simulink model "pendulum"  (Simulink 5.0)
settings: Solver=ode45  StartTime=0.00  StopTime=15  FixedStep=0.1  MaxStep=0.001  RelTol=1e-3
values from neighbouring files (symbols this model uses):
  K = [0 K]    [Pendulum_init.m]
libraries: vrlib x1
CloseFcn:
  | rtwprivate ssgencode ModelCloseRequest pendsim
settings Model: LastModifiedBy=Gato  RTWOptions="-aEnforceIntegerDowncast=1 -aExtMode=0 -aExtModeTesting=0 -aFoldNonRolledExpr=1 -aForceParamTrailComments=0 -aGenerateComments=1 -aGenerateReport=0 -aIgnoreCustomStorageClasses=1 -aIncDataTypeInIds=0 -aIncHierarchyInIds=0 -aInlineInvariantSignals=0 -aInlinedPrmAccess=\"Literals\" -aLocalBlockOutputs=1 -aLogVarNameModifier=\"rt_\" -aMaxRTWIdLen=31 -aPrefixModelToSubsysFcnNames=1 -aRTWVerbose=1 -aRollThreshold=5 -aShowEliminatedStatements=0"

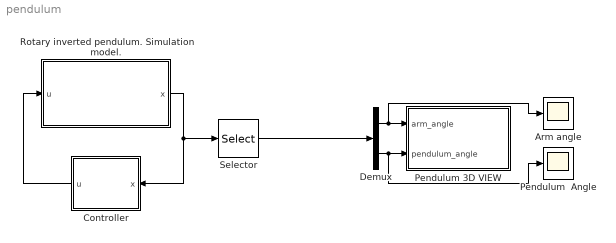
== system pendulum ==
  Arm angle : Scope
  Controller : Subsystem  Orientation=left
  Demux : Demux  Outputs=2
  Pendulum  Angle : Scope
  Pendulum 3D VIEW : Subsystem  TreatAsAtomicUnit=on
  Rotary inverted pendulum. Simulation model. : Subsystem  TreatAsAtomicUnit=on  mask{l=0.5, m1=1, b1=0.4, r=1, m2=0.5, b2=0.1, x1_0=0, x2_0=0, x3_0=0.1, x4_0=0, g=9.81}
      mask prompts: l "Arm length [m]"; m1 "Arm mass [kg]"; b1 "Arm dumping coefficient"; r "Pendulum lenght [m]"; m2 "Pendulum mass [kg]"; b2 "Pendulum dumping coefficient"; x1_0 "Arm initial angle [rad]"; x2_0 "Arm initial speed [m/s]"; x3_0 "Pendulum initial angle [rad]"; x4_0 "Pendulum initial speed [m/s]"; g "Gravity"
  Selector : Selector  Elements=[1 3]  InputPortWidth=4
  wires:
  Demux/1 -> Pendulum 3D VIEW/1(arm_angle), Arm angle/1
  Demux/2 -> Pendulum 3D VIEW/2(pendulum_angle), Pendulum  Angle/1
  Selector/1 -> Demux/1
  Rotary inverted pendulum. Simulation model./1(x) -> Selector/1, Controller/1(x)
  Controller/1(u) -> Rotary inverted pendulum. Simulation model./1(u)

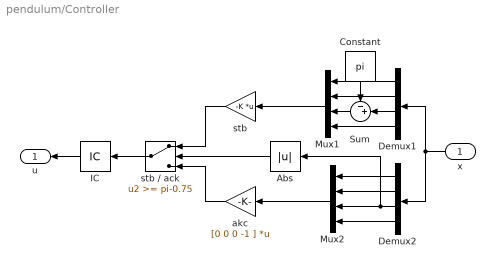
== system pendulum/Controller ==
  x : Inport  Orientation=left
  Abs : Abs  Orientation=left  SaturateOnIntegerOverflow=on
  Constant : Constant  Orientation=down  Value=pi
  Demux1 : Demux  Orientation=left
  Demux2 : Demux  Orientation=left
  IC : InitialCondition  Orientation=left  Value=0
  Mux1 : Mux  Orientation=left
  Mux2 : Mux  Orientation=left
  Sum : Sum  Orientation=left  Inputs=-+|  SaturateOnIntegerOverflow=on
  akc : Gain  Orientation=left  Gain=[0 0 0 -1 ]  Multiplication=Matrix(K*u)  SaturateOnIntegerOverflow=on
  stb : Gain  Orientation=left  Gain=-K  Multiplication=Matrix(K*u)  SaturateOnIntegerOverflow=on
  stb / ack : Switch  Orientation=left  Threshold=pi-0.75  SaturateOnIntegerOverflow=on
  u : Outport  Orientation=left
  wires:
  Demux2/2 -> Mux2/2
  Demux2/4 -> Mux2/4
  Demux2/1 -> Mux2/1
  Demux2/3 -> Mux2/3, Abs/1
  Mux2/1 -> akc/1
  IC/1 -> u/1
  Demux1/2 -> Mux1/2
  Demux1/1 -> Mux1/1
  stb/1 -> stb / ack/1
  Demux1/3 -> Sum/2
  Constant/1 -> Sum/1
  Sum/1 -> Mux1/3
  Mux1/1 -> stb/1
  Demux1/4 -> Mux1/4
  x/1 -> Demux1/1, Demux2/1
  akc/1 -> stb / ack/3
  Abs/1 -> stb / ack/2
  stb / ack/1 -> IC/1

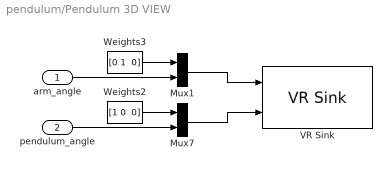
== system pendulum/Pendulum 3D VIEW ==
  arm_angle : Inport
  pendulum_angle : Inport  Port=2
  Mux1 : Mux  Inputs=2
  Mux7 : Mux  Inputs=2
  VR Sink : vrlib/VR Sink  SampleTime=0.1  ViewEnable=on  RemoteChange=off  RemoteView=off  FieldsWritten=Arm.rotation.4#Pendulum.rotation.4  WorldFileName=pendulum_vr.WRL  WorldDescription=pendulum_vr  AutoView=on  FigureProperties="{'Position', 'Name', 'Viewpoint', 'CameraBound', 'CameraDirection', 'CameraPosition', 'CameraUpVector', 'ZoomFactor', 'Antialiasing', 'Headlight', 'Lighting', 'PanelMode', 'Textures', 'Transparency', 'Wireframe', 'NavZones', 'InfoStrip', 'NavMode', 'NavSpeed', ; [9.0000000000000000e+000  2.5000000000000000e+001  6.5400000000000000e+002  9.6500000000000000e+002], 'pendulum_vr', '', 'on', [0.0000000000000000e+000  0.0000000000000000e+000 -1.0000000000000000e+000], [0.0000000000000000e+000  0.0000000000000000e+000  1.0000000000000000e+001], [0.0000000000000000e+000  1.0000000000000000e+000  0.0000000000000000e+000], [1.0000000000000000e+000], 'off', 'on', 'on', 'opaque', 'on', 'on', 'off', 'off', 'off', 'fly', 'normal', ; }"
  Weights2 : Constant  Value="[1 0  0]"
  Weights3 : Constant  Value="[0 1  0]"
  wires:
  Weights2/1 -> Mux7/1
  Mux7/1 -> VR Sink/2
  pendulum_angle/1 -> Mux7/2
  Weights3/1 -> Mux1/1
  Mux1/1 -> VR Sink/1
  arm_angle/1 -> Mux1/2

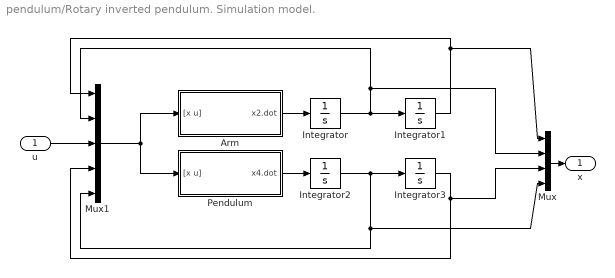
== system pendulum/Rotary inverted pendulum. Simulation model. ==
  u : Inport
  Arm : Subsystem  TreatAsAtomicUnit=on
  Integrator : Integrator  InitialCondition=x2_0
  Integrator1 : Integrator  InitialCondition=x1_0
  Integrator2 : Integrator  InitialCondition=x4_0
  Integrator3 : Integrator  InitialCondition=x3_0
  Mux : Mux
  Mux1 : Mux  Inputs=5
  Pendulum : Subsystem  TreatAsAtomicUnit=on
  x : Outport
  wires:
  Integrator3/1 -> Mux1/4, Mux/3
  Integrator2/1 -> Integrator3/1, Mux1/5, Mux/4
  Integrator/1 -> Integrator1/1, Mux1/2, Mux/2
  Pendulum/1(x4.dot) -> Integrator2/1
  Arm/1(x2.dot) -> Integrator/1
  Mux1/1 -> Pendulum/1("[x u]"), Arm/1("[x u]")
  u/1 -> Mux1/3
  Integrator1/1 -> Mux1/1, Mux/1
  Mux/1 -> x/1

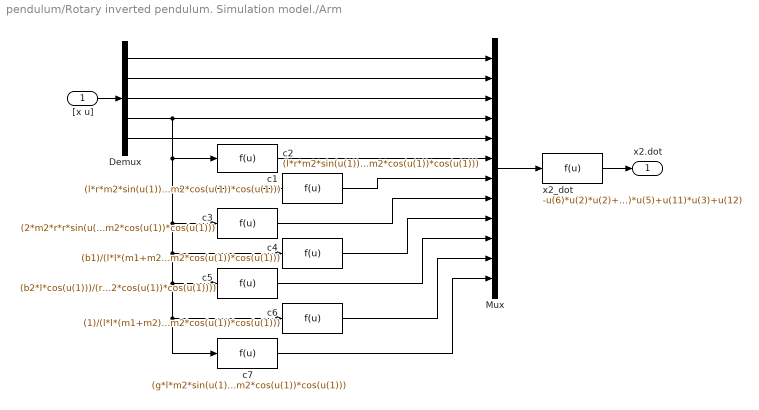
== system pendulum/Rotary inverted pendulum. Simulation model./Arm ==
  "[x u]" : Inport
  Demux : Demux  Outputs=5
  Mux : Mux  Inputs=12
  c1 : Fcn  Expr=(l*r*m2*sin(u(1))*cos(u(1))*cos(u(1)))/(l*l*(m1+m2)+r*r*m2*sin(u(1))*sin(u(1))-l*l*m2*cos(u(1))*cos(u(1)))
  c2 : Fcn  Expr=(l*r*m2*sin(u(1)))/(l*l*(m1+m2)+r*r*m2*sin(u(1))*sin(u(1))-l*l*m2*cos(u(1))*cos(u(1)))
  c3 : Fcn  Expr=(2*m2*r*r*sin(u(1))*cos(u(1)))/(l*l*(m1+m2)+r*r*m2*sin(u(1))*sin(u(1))-l*l*m2*cos(u(1))*cos(u(1)))
  c4 : Fcn  Expr=(b1)/(l*l*(m1+m2)+r*r*m2*sin(u(1))*sin(u(1))-l*l*m2*cos(u(1))*cos(u(1)))
  c5 : Fcn  Expr=(b2*l*cos(u(1)))/(r*(l*l*(m1+m2)+r*r*m2*sin(u(1))*sin(u(1))-l*l*m2*cos(u(1))*cos(u(1))))
  c6 : Fcn  Expr=(1)/(l*l*(m1+m2)+r*r*m2*sin(u(1))*sin(u(1))-l*l*m2*cos(u(1))*cos(u(1)))
  c7 : Fcn  Expr=(g*l*m2*sin(u(1))*cos(u(1)))/(l*l*(m1+m2)+r*r*m2*sin(u(1))*sin(u(1))-l*l*m2*cos(u(1))*cos(u(1)))
  x2_dot : Fcn  Expr=-u(6)*u(2)*u(2)+u(7)*u(5)*u(5)-u(8)*u(2)*u(5)-u(9)*u(2)+u(10)*u(5)+u(11)*u(3)+u(12)
  x2.dot : Outport
  wires:
  x2_dot/1 -> x2.dot/1
  c7/1 -> Mux/12
  c6/1 -> Mux/11
  c5/1 -> Mux/10
  c4/1 -> Mux/9
  c3/1 -> Mux/8
  c2/1 -> Mux/7
  c1/1 -> Mux/6
  Demux/5 -> Mux/5
  Demux/4 -> c1/1, c2/1, c3/1, c4/1, c6/1, c7/1, c5/1, Mux/4
  Demux/3 -> Mux/3
  Demux/2 -> Mux/2
  Demux/1 -> Mux/1
  Mux/1 -> x2_dot/1
  "[x u]"/1 -> Demux/1

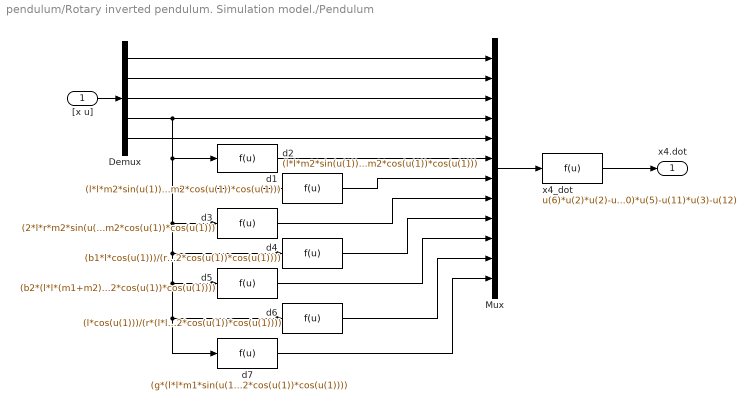
== system pendulum/Rotary inverted pendulum. Simulation model./Pendulum ==
  "[x u]" : Inport
  Demux : Demux  Outputs=5
  Mux : Mux  Inputs=12
  d1 : Fcn  Expr=(l*l*m2*sin(u(1))*cos(u(1))+l*l*m2*sin(u(1))*cos(u(1))+r*r*m2*sin(u(1))*sin(u(1))*sin(u(1))*cos(u(1)))/(l*l*(m1+m2)+r*r*m2*sin(u(1))*sin(u(1))-l*l*m2*cos(u(1))*cos(u(1)))
  d2 : Fcn  Expr=(l*l*m2*sin(u(1))*cos(u(1)))/(l*l*(m1+m2)+r*r*m2*sin(u(1))*sin(u(1))-l*l*m2*cos(u(1))*cos(u(1)))
  d3 : Fcn  Expr=(2*l*r*m2*sin(u(1))*cos(u(1)))/(l*l*(m1+m2)+r*r*m2*sin(u(1))*sin(u(1))-l*l*m2*cos(u(1))*cos(u(1)))
  d4 : Fcn  Expr=(b1*l*cos(u(1)))/(r*(l*l*(m1+m2)+r*r*m2*sin(u(1))*sin(u(1))-l*l*m2*cos(u(1))*cos(u(1))))
  d5 : Fcn  Expr=(b2*(l*l*(m1+m2)+r*r*m2*sin(u(1))*sin(u(1))))/(m2*r*r*(l*l*(m1+m2)+r*r*m2*sin(u(1))*sin(u(1))-l*l*m2*cos(u(1))*cos(u(1))))
  d6 : Fcn  Expr=(l*cos(u(1)))/(r*(l*l*(m1+m2)+r*r*m2*sin(u(1))*sin(u(1))-l*l*m2*cos(u(1))*cos(u(1))))
  d7 : Fcn  Expr=(g*(l*l*m1*sin(u(1))+l*l*m2*sin(u(1))+r*r*m2*sin(u(1))*sin(u(1))*sin(u(1))))/(r*(l*l*(m1+m2)+r*r*m2*sin(u(1))*sin(u(1))-l*l*m2*cos(u(1))*cos(u(1))))
  x4_dot : Fcn  Expr=u(6)*u(2)*u(2)-u(7)*u(5)*u(5)+u(8)*u(2)*u(5)+u(9)*u(2)-u(10)*u(5)-u(11)*u(3)-u(12)
  x4.dot : Outport
  wires:
  x4_dot/1 -> x4.dot/1
  d7/1 -> Mux/12
  d6/1 -> Mux/11
  d5/1 -> Mux/10
  d4/1 -> Mux/9
  d3/1 -> Mux/8
  d2/1 -> Mux/7
  d1/1 -> Mux/6
  Demux/5 -> Mux/5
  Demux/4 -> d1/1, d2/1, d3/1, d4/1, d5/1, d6/1, d7/1, Mux/4
  Demux/3 -> Mux/3
  Demux/2 -> Mux/2
  Demux/1 -> Mux/1
  Mux/1 -> x4_dot/1
  "[x u]"/1 -> Demux/1
